simulink model "Assignment_model3"  (R2015b)
settings: Solver=ode45  StartTime=0.0  StopTime=50  RelTol=1e-3
settings Model: Creator=Administrator  LastModifiedBy=raghavv
settings DataIOCC: SaveFormat=Array
settings DebuggingCC: SolverPrmCheckMsg=warning
settings HardwareCC: ProdBitPerPointer=32  ProdLargestAtomicFloat=None  ProdIntDivRoundTo=Undefined  ProdEndianess=Unspecified  ProdWordSize=32  ProdHWDeviceType=32-bit Generic
settings GRTTargetCC: GeneratePreprocessorConditionals=Disable all
settings ConfigComp: CovModelRefEnable=Off  CovSFcnEnable=off

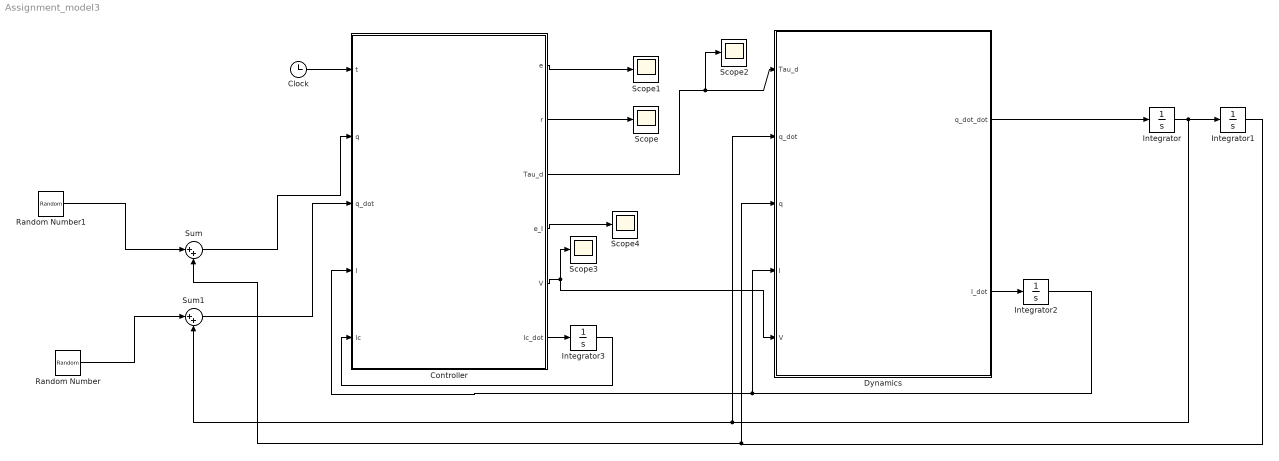
== system Assignment_model3 ==
  Clock : Clock
      settings: Decimation=50
  Controller : MATLAB Function  TreatAsAtomicUnit=on
  Dynamics : MATLAB Function  TreatAsAtomicUnit=on
  Integrator : Integrator  InitialCondition=[1;-1]
  Integrator1 : Integrator  InitialCondition=[1,9]
  Integrator2 : Integrator  InitialCondition=[0;0]
  Integrator3 : Integrator  InitialCondition=[0;0]
  Random Number : RandomNumber  Variance=0  SampleTime=0.1
  Random Number1 : RandomNumber  Variance=0  SampleTime=0.1
  Scope{,1..4} (5 alike) : Scope
  Sum : Sum  Inputs=|++
  Sum1 : Sum  Inputs=|++
  wires:
  Dynamics/1(q_dot_dot) -> Integrator/1
  Integrator/1 -> Integrator1/1, Sum1/2, Dynamics/2(q_dot)
  Integrator1/1 -> Sum/2, Dynamics/3(q)
  Clock/1 -> Controller/1(t)
  Random Number/1 -> Sum1/1
  Sum1/1 -> Controller/3(q_dot)
  Random Number1/1 -> Sum/1
  Controller/2(r) -> Scope/1
  Controller/1(e) -> Scope1/1
  Integrator2/1 -> Dynamics/4(I), Controller/4(I)
  Dynamics/2(I_dot) -> Integrator2/1
  Controller/3(Tau_d) -> Scope2/1, Dynamics/1(Tau_d)
  Sum/1 -> Controller/2(q)
  Controller/4(e_I) -> Scope4/1
  Controller/5(V) -> Dynamics/5(V), Scope3/1
  Controller/6(Ic_dot) -> Integrator3/1
  Integrator3/1 -> Controller/5(Ic)

== matlab function Assignment_model3/Controller ==
  data: e output; r output; Tau_d output; t input; q input; q_dot input; e_I output; I input; V output; Ic_dot output; Ic input
function [e,r,Tau_d,e_I,V,Ic_dot] = controller(t,q,q_dot,I,Ic) 

c2=cos(q(2));
s2=sin(q(2));
alpha=0.5;
k=0.5;

p1=3.473;
p2=0.196;
p3=0.242;
fd1=5.3;
fd2=1.1;

qd=[5*sin(t);10*cos(t)];
qd_dot=[5*cos(t);-10*sin(t)];
qd_ddot=[-5*sin(t);-10*cos(t)];
e=q-qd;     %Tracking Error
e_dot=q_dot-qd_dot;

r=e_dot+alpha*e;         %Filtered Tracking Error

%----------------------------------------------------------%
M=[p1+2*p3*c2 p2+p3*c2;p2+p3*c2 p2];% Inertia matrix
Vm=[-p3*s2*q_dot(2) -p3*s2*(q_dot(1)+q_dot(2));p3*s2*q_dot(1) 0];%Centripetal coriolis matrix
fd=[fd1 0;0 fd2]; % Friction matrix

Tau_d =-k*r+Vm*q_dot+fd*q_dot+M*qd_ddot-alpha*M*e_dot-Vm*r-e;         % Controller

c2_dot = -s2*q_dot(2);
s2_dot = c2*q_dot(2);

q_ddot=-M\(Vm*q_dot+fd*q_dot-Tau_d);

qd_ddot=[-5*sin(t);-10*cos(t)];
qd_dddot = [-5*cos(t);+10*sin(t)];
e_ddot=q_ddot-qd_ddot;

r_dot=e_ddot+alpha*e_dot;

Id = Tau_d;
M_dot =[2*p3*c2_dot p3*c2_dot;p3*c2_dot 0];
Vm_dot=[-p3*(s2*q_ddot(2)+s2_dot*q_dot(2)) -p3*(s2*(q_ddot(1)+q_ddot(2))+s2_dot*(q_dot(1)+q_dot(2)));p3*(s2*q_ddot(1)+s2_dot*q_dot(1)) 0];
%Vm_dot=[-p3*(s2_dot*q_dot(2)) -p3*(s2_dot*(q_dot(1)+q_dot(2)));p3*(s2_dot*q_dot(1)) 0];
%Id_dot=-k*(-qd_ddot+alpha*e_dot)+Vm_dot*q_dot+M_dot*qd_ddot+M*qd_dddot-alpha*(-M*qd_ddot-M_dot*e_dot)-Vm_dot*r-Vm*(-qd_ddot + alpha*e_dot) - e_dot;
Id_dot=-k*(r_dot)+Vm*q_ddot+Vm_dot*q_dot+fd*q_ddot+M_dot*qd_ddot+M*qd_dddot-alpha*(M*e_ddot+M_dot*e_dot)-Vm_dot*r-Vm*(r_dot) - e_dot;
e_I = I - Ic;
gamma = 0.01;
Ic_dot = (1/gamma)*(-Ic + Id);

V = q_dot + Ic_dot-(-Id) - r;

== matlab function Assignment_model3/Dynamics ==
  data: Tau_d input; q_dot_dot output; q_dot input; q input; I input; V input; I_dot output
function [q_dot_dot,I_dot]  = dynamics(Tau_d,q_dot,q, I, V)
%#codegen
p1=3.473;
p2=0.196;
p3=0.242;
fd1=5.3;
fd2=1.1;

c2=cos(q(2));
s2=sin(q(2));
% alpha=1;

M=[p1+2*p3*c2 p2+p3*c2;p2+p3*c2 p2];% Inertia matrix
Vm=[-p3*s2*q_dot(2) -p3*s2*(q_dot(1)+q_dot(2));p3*s2*q_dot(1) 0];%Centripetal coriolis matrix
fd=[fd1 0;0 fd2]; % Friction matrix
q_dot_dot=-M\(Vm*q_dot+fd*q_dot-Tau_d);   %EL dynamics

%as L = I2, inv(L) = I2;
I_dot = V - q_dot - I;
